simulink model "calculator"  (R2017a)
settings: Solver=FixedStepAuto  StartTime=0.0  StopTime=10  RelTol=1e-3  EnableMultiTasking=on
settings Model: Creator=Vincent  LastModifiedBy=Vincent
settings SolverCC: PositivePriorityOrder=on
settings OptimizationCC: PassReuseOutputArgsThreshold=0  MaxStackSize=64
settings DebuggingCC: ParameterTunabilityLossMsg=error
settings HardwareCC: ProdBitPerPointer=32  ProdBitPerSizeT=32  ProdBitPerPtrDiffT=32  ProdLargestAtomicInteger=Long  ProdLargestAtomicFloat=Double  ProdWordSize=32  ProdHWDeviceType=ARM Compatible->ARM Cortex  UseEmbeddedCoderFeatures=off
settings SFSimCC: MATLABDynamicMemAlloc=off
settings RTWCC: SystemTargetFile=ert.tlc  HardwareBoard=Raspberry Pi  TLCOptions="-aInlineSetEventsForThisBaseRateFcn=TLC_FALSE -aSuppressMultiTaskScheduler=TLC_FALSE  -aRateBasedStepFcn=0"  TemplateMakefile=ert_default_tmf  Description=Embedded Coder  GenerateReport=on  Toolchain=GNU GCC Raspberry Pi  LaunchReport=on
settings CodeAppCC: ForceParamTrailComments=on  OperatorAnnotations=on  MATLABSourceComments=on
settings ERTTargetCC: ERTCustomFileBanners=off  SupportContinuousTime=on  SupportNonInlinedSFcns=on  RemoveResetFunc=off  SupportVariableSizeSignals=on  ModelStepFunctionPrototypeControlCompliant=off

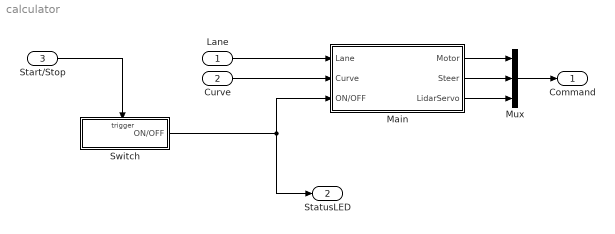
== system calculator ==
  Lane : Inport
  Curve : Inport  Port=2
  Start/Stop : Inport  Port=3
  Main : Subsystem  TreatAsAtomicUnit=on
  Mux : Mux  Inputs=3
  Switch : Subsystem  TreatAsAtomicUnit=on
  Command : Outport
  StatusLED : Outport  Port=2
  wires:
  Switch/1(ON/OFF) -> Main/3(ON/OFF), StatusLED/1
  Lane/1 -> Main/1(Lane)
  Curve/1 -> Main/2(Curve)
  Main/1(Motor) -> Mux/1
  Main/2(Steer) -> Mux/2
  Main/3(LidarServo) -> Mux/3
  Mux/1 -> Command/1
  Start/Stop/1 -> Switch/Trigger

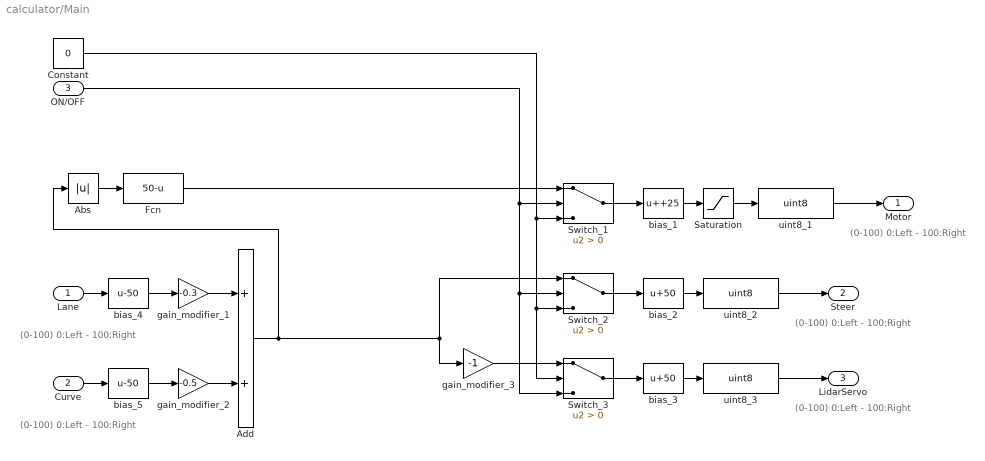
== system calculator/Main ==
  note: (0-100)
      | 0:Left - 100:Right
  note: (0-100)
      | 0:Left - 100:Right
  note: (0-100)
      | 0:Left - 100:Right
  note: (0-100)
      | 0:Left - 100:Right
  note: (0-100)
      | 0:Left - 100:Right
  Lane : Inport
  Curve : Inport  Port=2
  ON/OFF : Inport  Port=3
  Abs : Abs
  Add : Sum
  Constant : Constant  Value=0
  Fcn : Fcn  Expr=50-u
  Saturation : Saturate  UpperLimit=100  LowerLimit=60
  Switch_1 : Switch  Criteria=u2 > Threshold
  Switch_2 : Switch  Criteria=u2 > Threshold
  Switch_3 : Switch  Criteria=u2 > Threshold
  bias_1 : Bias  Bias=+25
  bias_2 : Bias  Bias=50
  bias_3 : Bias  Bias=50
  bias_4 : Bias  Bias=-50
  bias_5 : Bias  Bias=-50
  gain_modifier_1 : Gain  Gain=-0.3
  gain_modifier_2 : Gain  Gain=-0.5
  gain_modifier_3 : Gain  Gain=-1
  uint8_1 : DataTypeConversion  OutDataTypeStr=uint8
  uint8_2 : DataTypeConversion  OutDataTypeStr=uint8
  uint8_3 : DataTypeConversion  OutDataTypeStr=uint8
  Motor : Outport
  Steer : Outport  Port=2
  LidarServo : Outport  Port=3
  wires:
  uint8_2/1 -> Steer/1
  uint8_3/1 -> LidarServo/1
  uint8_1/1 -> Motor/1
  bias_2/1 -> uint8_2/1
  bias_3/1 -> uint8_3/1
  Lane/1 -> bias_4/1
  Curve/1 -> bias_5/1
  ON/OFF/1 -> Switch_3/3, Switch_2/2, Switch_1/2
  Constant/1 -> Switch_3/2, Switch_2/3, Switch_1/3
  Switch_3/1 -> bias_3/1
  Switch_2/1 -> bias_2/1
  Switch_1/1 -> bias_1/1
  bias_4/1 -> gain_modifier_1/1
  bias_5/1 -> gain_modifier_2/1
  gain_modifier_1/1 -> Add/1
  gain_modifier_2/1 -> Add/2
  Add/1 -> Abs/1, gain_modifier_3/1, Switch_2/1
  Abs/1 -> Fcn/1
  Fcn/1 -> Switch_1/1
  bias_1/1 -> Saturation/1
  Saturation/1 -> uint8_1/1
  gain_modifier_3/1 -> Switch_3/1

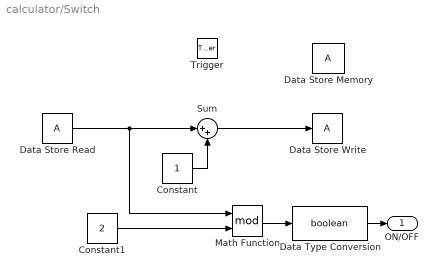
== system calculator/Switch ==
  Trigger : TriggerPort  VariantControl=Variant
  Constant : Constant
  Constant1 : Constant  Value=2
  Data Store Memory : DataStoreMemory  ReadBeforeWriteMsg=warning  WriteAfterWriteMsg=warning  WriteAfterReadMsg=warning  ShowAdditionalParam=off
  Data Store Read : DataStoreRead
  Data Store Write : DataStoreWrite
  Data Type Conversion : DataTypeConversion  OutDataTypeStr=boolean
  Math Function : Math  Operator=mod  SaturateOnIntegerOverflow=on
  Sum : Sum  Inputs=|++
  ON/OFF : Outport
  wires:
  Sum/1 -> Data Store Write/1
  Data Store Read/1 -> Math Function/1, Sum/1
  Constant/1 -> Sum/2
  Constant1/1 -> Math Function/2
  Math Function/1 -> Data Type Conversion/1
  Data Type Conversion/1 -> ON/OFF/1
